simulink model "Test9"  (R2021a)
settings: Solver=FixedStepDiscrete  StartTime=0.0  StopTime=tsim  FixedStep=Ts  RelTol=1e-3  EnableMultiTasking=on
InitFcn:
  | Fs = 2048; Ts = 1/Fs;tsim = inf;
undefined symbols (not defined in the file or in its folder): DiscIntNeverNeededParam
libraries: sperte_lib x24, simulink x5, Quintic_Polynomial_Trajectory_Library x3, raspberrypiCommlib x2
(part 2 of 2)

== system Test9/RobotArm/Supervisor/Supervisory Controller Z/Selector1 ==
  In1 : Inport
  Demux2 : Demux  Outputs=3
  Terminator4 : Terminator
  Terminator5 : Terminator
  Out1 : Outport
  wires:
  Demux2/3 -> Out1/1
  Demux2/2 -> Terminator5/1
  In1/1 -> Demux2/1
  Demux2/1 -> Terminator4/1

== system Test9/RobotArm/Supervisor/Supervisory Controller Z/Selector2 ==
  In1 : Inport
  Demux2 : Demux  Outputs=3
  Terminator4 : Terminator
  Terminator5 : Terminator
  Out1 : Outport
  wires:
  Demux2/1 -> Terminator4/1
  In1/1 -> Demux2/1
  Demux2/2 -> Terminator5/1
  Demux2/3 -> Out1/1

== system Test9/RobotArm/Supervisor/Supervisory Controller Z/Selector3 ==
  In1 : Inport
  Demux2 : Demux  Outputs=3
  Terminator5 : Terminator
  Out1 : Outport
  Out2 : Outport  Port=2
  wires:
  Demux2/3 -> Out1/1
  Demux2/2 -> Terminator5/1
  In1/1 -> Demux2/1
  Demux2/1 -> Out2/1

== system Test9/RobotArm/Supervisor/Supervisory Conveyor/Controller Conveyor ==
  Input : Inport
  Dct1lowpass : sperte_lib/Dct1lowpass  f_den=30
      settings: SourceProductName=SPERTE project library
  Dctintegrator3 : S-Function  FunctionName=dweakint  Parameters=f_num, 0.001  SFunctionDeploymentMode=off  EnableBusSupport=off  mask(dctools){f_num=0.01}
      mask prompts: f_num "Zero [Hz]"
      mask help: This block implements a discrete time weak integrator filter.
      mask Display: disp('DCT integrator')
  Dctleadlag : sperte_lib/Dctleadlag  f_num=3  f_den=20
      settings: SourceProductName=SPERTE project library
  Gain1 : Gain  Gain=10*2.5/500
  Output : Outport
  wires:
  Input/1 -> Gain1/1
  Dctintegrator3/1 -> Dct1lowpass/1
  Dctleadlag/1 -> Output/1
  Gain1/1 -> Dctintegrator3/1
  Dct1lowpass/1 -> Dctleadlag/1

== system Test9/RobotArm/Supervisor/Subsystem/LED Ring/Subsystem ==
  note: U(k)
  note: Edge
  U : Inport
  Delay : Delay  DelayLength=1  InitialCondition=0
  NOT : Logic  Operator=NOT  IconShape=distinctive  AllPortsSameDT=off  OutDataTypeStr=boolean
  String Compare : StringCompare
  Y : Outport  InitialOutput=0
  wires:
  Delay/1 -> String Compare/2  "U(k-1)"
  String Compare/1 -> NOT/1
  NOT/1 -> Y/1
  U/1 -> Delay/1, String Compare/1

== system Test9/RobotArm/Supervisor/Subsystem/LED Ring/Subsystem3 ==
  In1 : Inport
  Enable : EnablePort
  If : If  IfExpression=u1 == 1
  If Action Subsystem : Subsystem  TreatAsAtomicUnit=on
  If Action Subsystem1 : Subsystem  TreatAsAtomicUnit=on
  OR : Logic  Operator=OR  IconShape=distinctive  AllPortsSameDT=off  OutDataTypeStr=boolean
  String Compare : StringCompare
  String Compare1 : StringCompare
  String Constant1 : StringConstant  String='black'
  String Constant4 : StringConstant  String='white'
  wires:
  If/1 -> If Action Subsystem/Action
  String Compare/1 -> OR/1
  String Constant4/1 -> String Compare/2
  In1/1 -> If Action Subsystem1/1(In1), String Compare1/1, String Compare/1, If Action Subsystem/1(In1)
  If/2 -> If Action Subsystem1/Action
  OR/1 -> If/1
  String Compare1/1 -> OR/2
  String Constant1/1 -> String Compare1/2

== system Test9/RobotArm/Supervisor/Subsystem/LED Ring/Subsystem3/If Action Subsystem ==
  In1 : Inport
  Action Port : ActionPort  ActionPortLabel=if(u1 == 1)
  Constant1 : Constant  Value=13  OutDataTypeStr=uint8
  Matrix Concatenate1 : Concatenate  ConcatenateDimension=2
  Serial Write1 : raspberrypiCommlib/Serial Write  board=Pi 4 Model B  SCIModule_=/dev/ttyACM0  Baudrate_=9600  Parity=None  StopBits_=1  HardwareFlowControl=None  ByteOrder=LittleEndian  OutputStatus=off  blockPlatform=RaspberryPi
      settings: SourceProductBaseCode=RASPPI
  String to ASCII1 : StringToASCII
  wires:
  In1/1 -> String to ASCII1/1
  String to ASCII1/1 -> Matrix Concatenate1/1
  Matrix Concatenate1/1 -> Serial Write1/1
  Constant1/1 -> Matrix Concatenate1/2

== system Test9/RobotArm/Supervisor/Subsystem/LED Ring/Subsystem3/If Action Subsystem1 ==
  In1 : Inport
  Action Port : ActionPort  ActionPortLabel=else
  Constant : Constant  Value=13  OutDataTypeStr=uint8
  Matrix Concatenate : Concatenate  ConcatenateDimension=2
  Serial Write : raspberrypiCommlib/Serial Write  board=Pi 4 Model B  SCIModule_=/dev/ttyACM0  Baudrate_=9600  Parity=None  StopBits_=1  HardwareFlowControl=None  ByteOrder=LittleEndian  OutputStatus=off  blockPlatform=RaspberryPi
      settings: SourceProductBaseCode=RASPPI
  String Concatenate : StringConcatenate
  String Constant3 : StringConstant  String='color '
  String to ASCII : StringToASCII
  wires:
  Matrix Concatenate/1 -> Serial Write/1
  String to ASCII/1 -> Matrix Concatenate/1
  String Concatenate/1 -> String to ASCII/1
  String Constant3/1 -> String Concatenate/1
  Constant/1 -> Matrix Concatenate/2
  In1/1 -> String Concatenate/2

== matlab function Test9/RobotArm/Supervisor/Supervisory Controller R/Angle2Z ==
  data: u input; y output
function y = fcn(u)

% Z and X angles to height of the robotarm. The initial angles are the
% angles from the horizontal line to the correponding arm.

initialanglez = 0.6150;
initialanglex = (75.3841/180)*pi;
thetax = -u(2)+initialanglex;
thetaz = u(3)+initialanglez;

theta1 = thetax;
theta2 = thetaz;

% parameters

l1 = 80e-3;
l2 = 130e-3;
l3 = 165e-3;
l4 = 130e-3;
l5 = 120e-3;
l6 = 120e-3 + 65e-3;
length_head = 45e-3;
l7 = 81e-3;

% functions

fx1 = l1*cos(theta1);
fy1 = l1*sin(theta1);

fx2 = l2*cos(theta2);
fy2 = l3 + l2*sin(theta2);

d12 = sqrt((fx2 - fx1)^2 + (fy2 - fy1)^2);
d13 = sqrt(fx1^2 + (l3 - fy1)^2);

phi1 = acos((l2^2 + d12^2 -d13^2)/(2*d12*l2));
phi2 = acos((l5^2 + d12^2 -l4^2)/(2*d12*l5));

yf = fy2- l6*sin(pi - phi1 - phi2 - theta2);

y = yf-length_head+l7;

== matlab function Test9/RobotArm/Supervisor/Supervisory Controller Z/Angle2Z ==
  data: u input; y output
function y = fcn(u)

% Z and X angles to height of the robotarm. The initial angles are the
% angles from the horizontal line to the correponding arm.

initialanglez = 0.6150;
initialanglex = (75.3841/180)*pi;
thetax = -u(2)+initialanglex;
thetaz = u(3)+initialanglez;

theta1 = thetax;
theta2 = thetaz;

% parameters

l1 = 80e-3;
l2 = 130e-3;
l3 = 165e-3;
l4 = 130e-3;
l5 = 120e-3;
l6 = 120e-3 + 65e-3;
length_head = 45e-3;
l7 = 81e-3;

% functions

fx1 = l1*cos(theta1);
fy1 = l1*sin(theta1);

fx2 = l2*cos(theta2);
fy2 = l3 + l2*sin(theta2);

d12 = sqrt((fx2 - fx1)^2 + (fy2 - fy1)^2);
d13 = sqrt(fx1^2 + (l3 - fy1)^2);

phi1 = acos((l2^2 + d12^2 -d13^2)/(2*d12*l2));
phi2 = acos((l5^2 + d12^2 -l4^2)/(2*d12*l5));

yf = fy2- l6*sin(pi - phi1 - phi2 - theta2);

y = yf-length_head+l7;

== stateflow chart Test9/Controller/Stateflow  ==
  settings: updateMethod=DISCRETE  sampleTime=0.00048828125  executeAtInitialization=1
  state Robot_Arm [parallel]
    settings: executionOrder=4
    state Start_Home
      entry:
      [R_rad, X_rad, Z_rad] = invkin(X_home, Y_home, Z_home); %Move to home
      WaitFor = TimeToMoveCalc(TimeBuffer, R_radVavg, X_radVavg, Z_radVavg, R_rad, X_rad, Z_rad, R_radMeasure, X_radMeasure, Z_radMeasure)
    state Await_Scanning
      entry:
      ScanAgain
      PumpOff
    state Move_TrackingAwaitingLocation
      entry:
      [R_rad, X_rad, Z_rad] = invkinBound(X_in, Y_StartMoveAlong , Z_StartMoveAlong);
      WaitFor = TimeToMoveCalc(TimeBuffer, R_radVavg, X_radVavg, Z_radVavg, R_rad, X_rad, Z_rad, R_radMeasure, X_radMeasure, Z_radMeasure)
    state Get_Data
      entry:
      Y_data = Y_in;
      X_data = X_in;
      Z_arm = Z_StartMoveAlong; %99 or Z_home
      Area_data = Area_in;
    state Move_TrackingAndPickUp
      entry:
      if (n<1)
      Y_obj = Y_data + (TimeStep+CameraDelay)*Conveyor;
      n = n+1;
      elseif (n>=1)
      Y_obj = Y_obj+(TimeStep)*Conveyor;
      %if Y_obj <= Y_StartMoveAlong %-60
      % [R_rad, X_rad, Z_rad] = invkinBound(X_data, Y_obj, Z_arm)
      if Y_obj > Y_StartLowering %-60
      Z_arm = Z_arm - abs(Z_StartMoveAlong-Z_PickUpHeight)/abs(Y_PickUpAt-Y_StartLowering)*Conveyor*TimeStep;
      [R_rad, X_rad, Z_rad] = invkinBound(X_data, Y_obj, Z_arm);
      if Z_arm <= Z_PickUpHeight % 80
      Tracking = false;
      send(VacuumOn,Pump_stateflow);
      end
      end
      end
    state Move_toGoalHeight1
      entry:
      Z_arm = Z_arm+18;
      [R_radt, X_radt, Z_radt] = invkinBound(X_data, Y_obj, Z_arm); %Move to goal xy at setpoint height
      WaitFor = TimeToMoveCalc(TimeBuffer, R_radVavg, X_radVavg, Z_radVavg, R_radt, X_radt, Z_radt, R_radMeasure, X_radMeasure, Z_radMeasure)
    state Move_toGoalHeight2
      entry:
      [R_radt, X_radt, Z_radt] = invkinBound(150, 60, Z_arm+2); %Move to goal xy at setpoint height
      WaitFor = TimeToMoveCalc(TimeBuffer, R_radVavg, X_radVavg, Z_radVavg, R_radt, X_radt, Z_radt, R_radMeasure, X_radMeasure, Z_radMeasure)
    state Move_toGoalLower
      entry:
      GetEndXY
      [R_rad, X_rad, Z_rad] = invkinBound(EndX, EndY, Z_arm+2); %Lower until ready to drop item
      WaitFor = TimeToMoveCalc(TimeBuffer, R_radVavg, X_radVavg, Z_radVavg, R_rad, X_rad, Z_rad, R_radMeasure, X_radMeasure, Z_radMeasure)
    state Eject_object
      entry:
      BlowOn
    (default) -> Start_Home
    (junction 408) -> Start_Home
    Eject_object -> (junction 408) : [VacuumSensor>-0.014]
    Start_Home -> Await_Scanning : [after(WaitFor,sec)]
    Await_Scanning -> Move_TrackingAwaitingLocation : [Area_in>=2000]
    Move_TrackingAwaitingLocation -> Get_Data : [(after(WaitFor, sec))&&(Y_in> -120)]{Tracking = true, n=0}
    Get_Data -> Move_TrackingAndPickUp
    Move_TrackingAndPickUp -> Move_TrackingAndPickUp [order 1] : [Tracking == true&&after(TimeStep,sec)]
    Move_TrackingAndPickUp -> Move_toGoalHeight1 [order 2] : [(Tracking==false)&&(VacuumSensor<-0.35)]
    Move_toGoalHeight1 -> Move_toGoalHeight2 : [after(WaitFor, sec)]
    Move_toGoalHeight2 -> Move_toGoalLower : [after(WaitFor, sec)]
    Move_toGoalLower -> Eject_object : [after(WaitFor, sec)]
  state Object_Detection [parallel]
    settings: executionOrder=1
    state Seeking
      entry:
    state AwaitSeeking
      entry:
      GetProduct
    state ProvideData
      entry:
      if (3000<=Area_data)&&(Area_data<6000)
      nPawn = nPawn + 1;
      EndX = 45-(nPawn-1)*48; % Pawn (a-h)2
      EndY = 193;
      elseif (6000<=Area_data)&&(Area_data<8600)
      EndX = -51; % Knight b1
      EndY = 145;
      elseif (8600<=Area_data)&&(Area_data<12000)
      EndX = -3; % Bishop c1
      EndY = 145;
      elseif (12000<=Area_data)&&(Area_data<15000)
      EndX = -98; % Rook a1
      EndY = 145;
      elseif (15000<=Area_data)&&(Area_data<17000)
      EndX = 45; % Queen d1
      EndY = 145;
      elseif (17000<=Area_data)&&(Area_data<27000)
      EndX = 45; % King d1 (there is no e1)
      EndY = 145;
      end
    (default) -> Seeking
    (junction 428) -> Seeking
    (junction 448) -> (junction 428)
    Seeking -> AwaitSeeking : [Area_in>=2000]
    AwaitSeeking -> ProvideData : GetEndXY
    ProvideData -> (junction 448) : ScanAgain
  state Pump_stateflow [parallel]
    settings: executionOrder=3
    state Pump_off
      during:
      Pump = 0 %Bar
      Blow_suck = 1
    state Vacuum
      during:
      Pump = -1 %Bar
      Blow_suck = 0
    state Blow
      during:
      Pump = 1 %Bar
      Blow_suck = 1
    (default) -> Pump_off
    Pump_off -> Vacuum [order 1] : VacuumOn
    Vacuum -> Pump_off [order 1] : PumpOff
    Blow -> Pump_off [order 2] : PumpOff
    Pump_off -> Blow [order 2] : BlowOn
    Blow -> Vacuum [order 1] : VacuumOn
    Vacuum -> Blow [order 2] : BlowOn
  state Belt [parallel]
    settings: executionOrder=2
    state Belt_Home
      during:
      Conveyor = 30;
    (default) -> Belt_Home
  data: errorAngleDegree function_input; R_rad_GoTo function_input; X_rad_GoTo function_input; Z_rad_GoTo function_input; R_rad_Current function_input; X_rad_Current function_input; Z_rad_Current function_input; RXZ_OnPosition function_output; x_kin function_input; y_kin function_input; z_kin function_input; PsikinBound function_output; PhikinBound function_output; ThetakinBound function_output; x_kin function_input; y_kin function_input; z_kin function_input; Psikin function_output; Phikin function_output; Thetakin function_output; BufferTime function_input; Rrad_Vavg function_input; Xrad_Vavg function_input; Zrad_Vavg function_input; Rrad_goto function_input; Xrad_goto function_input; Zrad_goto function_input; Rrad_current function_input; Xrad_current function_input; Zrad_current function_input; MoveAfterXSec function_output; R_rad output; X_in input; X_rad output; Z_rad output; Y_in input; Area_in input; VacuumSensor input; Blow_suck output; Conveyor output; Pump output; Tracking output boolean =true; R_radMeasure input; X_radMeasure input; Z_radMeasure input; R_radVavg input; X_radVavg input; Z_radVavg input; WaitFor local; CameraDelay input; Y_StartMoveAlong local =-60; Y_StartLowering local =-60; Z_PickUpHeight local =80; X_home local =160; Y_home local =0; Z_home local =90; Z_StartMoveAlong local =90; Y_PickUpAt local =0; nPawn local =0; X_data local; Y_data local; EndX local; EndY local; TimeBuffer local =0.4; n local =0; TimeStep local =0.01; R_radt local; X_radt local; Z_radt local; Y_obj local =0; Z_arm local =90; Area_data local =0
  events: GetProduct local FUNCTION_CALL_EVENT; ScanAgain local FUNCTION_CALL_EVENT; VacuumOn local FUNCTION_CALL_EVENT; BlowOn local FUNCTION_CALL_EVENT; PumpOff local FUNCTION_CALL_EVENT; GetEndXY local RISING_EDGE_EVENT
  function RXZ_OnPosition = RXZOnPosition(errorAngleDegree, R_rad_GoTo, X_rad_GoTo, Z_rad_GoTo, R_rad_Current, X_rad_Current, Z_rad_Current):
    | function RXZ_OnPosition = RXZOnPosition(errorAngleDegree, R_rad_GoTo, X_rad_GoTo, Z_rad_GoTo, R_rad_Current, X_rad_Current, Z_rad_Current)
    | 
    | % Standard Output
    | OnPositionR = false;
    | OnPositionX = false;
    | OnPositionZ = false;
    | RXZ_OnPosition = false;
    | 
    | % Calculate error
    | R_error = abs(R_rad_Current-R_rad_GoTo);
    | X_error = abs(X_rad_Current-X_rad_GoTo);
    | Z_error = abs(Z_rad_Current-Z_rad_GoTo);
    | errorAngleRad = errorAngleDegree;
    | 
    | 
    | % Check if error is within a certain percentage of the current movement
    | if (R_error <= errorAngleRad)
    |     OnPositionR = true;
    | end
    | if (X_error <= errorAngleRad)
    |     OnPositionX = true;
    | end
    | if (X_error <= errorAngleRad)
    |     OnPositionZ = true;
    | end
    | % Return function as true when final coordinates are reached for all
    | if OnPositionR&&OnPositionX&&OnPositionZ
    |     RXZ_OnPosition = true;
    | end
    | 
    | 
    | end
  function [PsikinBound, PhikinBound, ThetakinBound] = invkinBound(x_kin, y_kin, z_kin):
    | function [PsikinBound, PhikinBound, ThetakinBound] = invkinBound(x_kin, y_kin, z_kin)
    | %% function to determine the angle of the motors for the right x,y,z position
    | %% Psi is angle R motor in rad
    | %% Phi is angle X motor in rad
    | %% Theta is angle Z motor in rad
    | %% x [mm] is perpendicular to the conveyer
    | %% y [mm] is in the direction of the conveyer
    | %% Z [mm]is the height from the conveyer
    | 
    | % These offsets are for the homing position (160, 0, 99) w.r.t. the middle
    | % of the robotarm on the table
    | r_offset = 0;
    | x_offset = -0.2551;
    | z_offset = -0.6150;
    | 
    | mm  = 10^(-3);
    | L1  = 130*mm;
    | L2a = 120*mm;
    | L2b = 65*mm;
    | L2  = L2a+L2b;
    | L3  = 80*mm;
    | L4  = 130*mm;
    | ED  = 165*mm;
    | OE  = 81*mm;
    | 
    | %% measurements
    | length_head = 45*mm;              % length of the vacuum head
    | height_conveyer = 0*mm;           % height of the conveyer
    | X0 = 0*mm;                        % distance center robot to conveyer
    | Y0      =   0*mm;                    % distance center plate to grid
    | 
    | %% Determine the x, y and z coordinates of the grid in [m]
    | Y = Y0+y_kin*mm;
    | X = X0+x_kin*mm;
    | Z = length_head+height_conveyer+z_kin*mm;
    | 
    | %% Psi - motor R
    | R   =   sqrt(X^2+Y^2);
    | PsikinBound =   atan2(Y,X);
    | 
    | %% Theta - motor Z
    | L_DB    = sqrt(R^2+(OE+ED-Z)^2);
    | H_GDB   = asin(R/L_DB);
    | H_CDB   = acos((L1^2+L_DB^2-L2^2)/(2*L1*L_DB));
    | ThetakinBound   = H_CDB+H_GDB-.5*pi;
    | 
    | %% PHI - motor X
    | H_DBC   = acos((L2^2+L_DB^2-L1^2)/(2*L2*L_DB));
    | H_DCB   = pi-H_CDB-H_DBC;
    | L_DF    = sqrt(L1^2+L2a^2-2*L1*L2a*cos(H_DCB));
    | H_CDF   = acos((L1^2+L_DF^2-L2a^2)/(2*L1*L_DF));
    | H_EDF   = H_CDB+H_GDB-H_CDF;
    | L_EF    = sqrt(L_DF^2+ED^2-2*L_DF*ED*cos(H_EDF));
    | H_DEF   = acos((L_EF^2+ED^2-L_DF^2)/(2*L_EF*ED));
    | Phi_2   = acos((L3^2+L_EF^2-L4^2)/(2*L3*L_EF));
    | Phi_1   = 0.5*pi-H_DEF;
    | PhikinBound     = Phi_1+Phi_2;
    | 
    | %% Final results of the angles
    | PsikinBound     = PsikinBound+r_offset;      % offset R
    | PhikinBound     = pi/2-PhikinBound+x_offset; % offset X
    | ThetakinBound   = ThetakinBound+z_offset;    % offset Z
    | 
    | % Check if answer is real, otherwise take sign of imaginary for rotation
    | % Set answer so it is real and definitely out of bounds, but with right sign 
    | if ~isreal(PsikinBound)
    | PsikinBound = sign(imag(PsikinBound))*6;
    | end
    | if ~isreal(PhikinBound)
    | PhikinBound = sign(imag(PhikinBound))*6;
    | end
    | if ~isreal(ThetakinBound)
    | ThetakinBound = sign(imag(ThetakinBound))*6;
    | end
    | 
    | % Check if angle is within bound, otherwise take the boundary
    | if ~((PsikinBound>-1)&&(PsikinBound<2))
    |     PsikinBound = min(max(PsikinBound,-1),2);
    | end
    | if ~((PhikinBound>-0.5)&&(PhikinBound<0.5))
    |     PhikinBound = min(max(PhikinBound,-0.5),0.5);
    | end
    | if ~((ThetakinBound>-0.3)&&(ThetakinBound<0.2))
    |     ThetakinBound = min(max(ThetakinBound,-0.3),0.2);
    | end
    | 
    | end
  function [Psikin, Phikin, Thetakin] = invkin(x_kin, y_kin, z_kin):
    | function [Psikin, Phikin, Thetakin] = invkin(x_kin, y_kin, z_kin)
    | %% function to determine the angle of the motors for the right x,y,z position
    | %% Psi is angle R motor in rad
    | %% Phi is angle X motor in rad
    | %% Theta is angle Z motor in rad
    | %% x [mm] is perpendicular to the conveyer
    | %% y [mm] is in the direction of the conveyer
    | %% Z [mm]is the height from the conveyer
    | 
    | % These offsets are for the homing position (160, 0, 99) w.r.t. the middle
    | % of the robotarm on the table
    | r_offset = 0;
    | x_offset = -0.2551;
    | z_offset = -0.6150;
    | 
    | mm  = 10^(-3);
    | L1  = 130*mm;
    | L2a = 120*mm;
    | L2b = 65*mm;
    | L2  = L2a+L2b;
    | L3  = 80*mm;
    | L4  = 130*mm;
    | ED  = 165*mm;
    | OE  = 81*mm;
    | 
    | %% measurements
    | length_head = 45*mm;              % length of the vacuum head
    | height_conveyer = 0*mm;           % height of the conveyer
    | X0 = 0*mm;                        % distance center robot to conveyer
    | Y0      =   0*mm;                    % distance center plate to grid
    | 
    | %% Determine the x, y and z coordinates of the grid in [m]
    | Y = Y0+y_kin*mm;
    | X = X0+x_kin*mm;
    | Z = length_head+height_conveyer+z_kin*mm;
    | 
    | %% Psi - motor R
    | R   =   sqrt(X^2+Y^2);
    | Psikin =   atan2(Y,X);
    | 
    | %% Theta - motor Z
    | L_DB    = sqrt(R^2+(OE+ED-Z)^2);
    | H_GDB   = asin(R/L_DB);
    | H_CDB   = acos((L1^2+L_DB^2-L2^2)/(2*L1*L_DB));
    | Thetakin   = H_CDB+H_GDB-.5*pi;
    | 
    | %% PHI - motor X
    | H_DBC   = acos((L2^2+L_DB^2-L1^2)/(2*L2*L_DB));
    | H_DCB   = pi-H_CDB-H_DBC;
    | L_DF    = sqrt(L1^2+L2a^2-2*L1*L2a*cos(H_DCB));
    | H_CDF   = acos((L1^2+L_DF^2-L2a^2)/(2*L1*L_DF));
    | H_EDF   = H_CDB+H_GDB-H_CDF;
    | L_EF    = sqrt(L_DF^2+ED^2-2*L_DF*ED*cos(H_EDF));
    | H_DEF   = acos((L_EF^2+ED^2-L_DF^2)/(2*L_EF*ED));
    | Phi_2   = acos((L3^2+L_EF^2-L4^2)/(2*L3*L_EF));
    | Phi_1   = 0.5*pi-H_DEF;
    | Phikin     = Phi_1+Phi_2;
    | 
    | %% Final results of the angles
    | Psikin     = Psikin+r_offset;      % offset R
    | Phikin     = pi/2-Phikin+x_offset; % offset X
    | Thetakin   = Thetakin+z_offset;    % offset Z
    | end
  function MoveAfterXSec = TimeToMoveCalc(BufferTime, Rrad_Vavg, Xrad_Vavg, Zrad_Vavg, Rrad_goto, Xrad_goto, Zrad_goto, Rrad_current, Xrad_current, Zrad_current):
    | function  MoveAfterXSec = TimeToMoveCalc(BufferTime, Rrad_Vavg, Xrad_Vavg, Zrad_Vavg, Rrad_goto, Xrad_goto, Zrad_goto, Rrad_current, Xrad_current, Zrad_current)
    | 
    | %TimeBuffer = 0.4; %sec
    | %Rrad_Vavg = 1;
    | %Xrad_Vavg = 1;
    | %Zrad_Vavg = 1;
    | %Rrad_goto = 2;
    | %Xrad_goto = 0.5;
    | %Zrad_goto = 0.2;
    | %Rrad_current = -1;
    | %Xrad_current = -0.5;
    | %Zrad_current = -0.3;
    | 
    | 
    | % t = delta_x/v_avg
    | Rrad_movetime = abs(Rrad_goto - Rrad_current)/Rrad_Vavg; 
    | Xrad_movetime = abs(Xrad_goto - Xrad_current)/Xrad_Vavg; 
    | Zrad_movetime = abs(Zrad_goto - Zrad_current)/Zrad_Vavg; 
    | 
    | 
    | 
    | MoveAfterXSec = BufferTime + max([Rrad_movetime, Xrad_movetime, Zrad_movetime]);
    | 
    | 
    | 
    | 
    | end

== stateflow chart Test9/RobotArm/Supervisor/Supervisory Conveyor/Supervisor ==
  state Waiting
    %Homing has to wait for 3 sec
    %as the new arm gets the 5V enable signal
    %after pressing start to avoi d moving to X0 too
    %early
  state Homing
    entry:
    %Set jog speed and homing state
    Ready=0;
    homingBusy = 1;
    jogSpeed = 20;
    homeControllerEnabled=1;
  state MovetoX0
    entry:
    jogSpeed = -20;
  state CheckRobotIsON
    entry:
    jogSpeed = 0;
  state WaitForRest
    entry: Ready = 1;
  state EnableRunAndSafety
    entry:
    resetEnc=0;
    homingBusy=0;
  state ResetEnc
    entry:
    resetEnc=1;
    homeControllerEnabled=0;
  (default) -> Waiting
  Waiting -> Homing : after(1,sec)
  Homing -> MovetoX0 : after(3,sec)
  MovetoX0 -> CheckRobotIsON : %Allow time for moving
      | after(3,sec)
  CheckRobotIsON -> WaitForRest : after(1,sec)
  WaitForRest -> ResetEnc : [AllReady]
  ResetEnc -> EnableRunAndSafety : after(1,sec)
  data: jogSpeed output double; homeControllerEnabled output double; resetEnc output double; homingBusy output double =1; Ready output double =1; AllReady input boolean; StopSim output double =0

== stateflow chart Test9/RobotArm/Supervisor/Supervisory Controller R/Supervisor ==
  state Waiting
    %Homing has to wait for 3 sec
    %as the new arm gets the 5V enable signal
    %after pressing start to avoid moving to X0 too
    %early
    Ready=0;
    toPoint = 0;
    homingBusy = 1;
    jogSpeed = -0.001;
    homeControllerEnabled=0.01;
  state Waiting1
    %Homing has to wait for 3 sec
    %as the new arm gets the 5V enable signal
    %after pressing start to avoid moving to X0 too
    %early
    Ready=0;
    toPoint = 0;
    homingBusy = 1;
    jogSpeed = 0;
    homeControllerEnabled=1;
  state AirbagLeft
    entry:
    homingBusy = 1;
    currentcarPos = carPos;
    airBagEnabled = 1;
    airBagRef=currentcarPos+0.02;
  state DisableOutputs
    entry:
    controlEnabled=0;
    StopSim = 1;
  state Homing
    entry:
    %Set jog speed and homing state
    Ready=0;
    toPoint = 0;
    homingBusy = 1;
    jogSpeed = -0.4;
    homeControllerEnabled=1;
  state AirbagLeft1
    entry:
    homingBusy = 1;
    currentcarPos = carPos;
    airBagEnabled = 1;
    airBagRef=currentcarPos-0.02;
  state AirbagConveyor
    entry:
    homingBusy = 1;
    currentcarPos = carPos;
    airBagEnabled = 1;
    airBagRef=currentcarPos+0.02
  state MovetoX0
    entry:
    jogSpeed = 0.0;
    toPoint = Offset_homing
  state STOPRobotIsOFF
    entry:
    StopSim=1;
  state CheckRobotIsON
  state EnableRunAndSafety
    entry:
    resetEnc=0;
    homingBusy=0;
  state RobotIsON
  state WaitForRest
    entry: Ready = 1;
  state ResetEnc
    entry:
    homingBusy = 100;
    resetEnc=1;
    homeControllerEnabled=0;
  (default) -> Waiting
  Waiting -> Waiting1 : after(1,sec)
  Waiting1 -> Homing : after(3,sec)
  AirbagLeft -> DisableOutputs : after(3,sec)
  AirbagConveyor -> DisableOutputs : after(3,sec)
  AirbagLeft1 -> DisableOutputs : after(3,sec)
  EnableRunAndSafety -> AirbagLeft [order 2] : [carPos<-1.1]
  Homing -> MovetoX0 : %Transition if homeswitch becomes high
      | [homeSwitch]
  EnableRunAndSafety -> AirbagLeft1 [order 1] : [carPos>2.7]
  EnableRunAndSafety -> AirbagConveyor [order 3] : [zcoordinate<0.056&&carPos < 1.3]
  MovetoX0 -> CheckRobotIsON [order 2] : % Allow time for moving
      | after(5,sec)
  MovetoX0 -> CheckRobotIsON [order 1] : [carPos == toPoint]
  CheckRobotIsON -> STOPRobotIsOFF [order 1] : [carPos<-3]
  CheckRobotIsON -> RobotIsON [order 2]
  RobotIsON -> WaitForRest : after(1,sec)
  ResetEnc -> EnableRunAndSafety : after(1,sec)
  WaitForRest -> ResetEnc : [AllReady]
  data: jogSpeed output double; toPoint output double; homeControllerEnabled output double; resetEnc output double; homingBusy output double =1; homeSwitch input boolean; carPos input double; airBagEnabled output double =0; airBagRef output double =0; controlEnabled output double =1; Ready output double =1; AllReady input boolean; StopSim output double =0; zcoordinate input; currentcarPos local double; Offset_homing input

== stateflow chart Test9/RobotArm/Supervisor/Supervisory Controller X/Supervisor ==
  state Waiting
    %Homing has to wait for 3 sec
    %as the new arm gets the 5V enable signal
    %after pressing start to avoid moving to X0 too
    %early
    Ready=0;
    toPoint = 0;
    homingBusy = 1;
    jogSpeed = -0.001;
    homeControllerEnabled=0.01;
  state DisableOutputs
    entry:
    controlEnabled=0;
    StopSim=1;
  state AirbagLeft
    entry:
    homingBusy = 1;
    currentcarPos = carPos;
    airBagEnabled = 1;
    airBagRef=currentcarPos+0.02;
  state Waiting1
    %Homing has to wait for 3 sec
    %as the new arm gets the 5V enable signal
    %after pressing start to avoid moving to X0 too
    %early
    Ready=0;
    toPoint = 0;
    homingBusy = 1;
    jogSpeed = 0;
    homeControllerEnabled=1;
  state AirbagRight
    entry:
    homingBusy = 1;
    currentcarPos = carPos;
    airBagEnabled = 1;
    airBagRef=currentcarPos-0.02;
  state Homing
    entry:
    %Set jog speed and homing state
    jogSpeed = -0.2;
    homeControllerEnabled=1;
  state MovetoX0
    entry:
    jogSpeed = 0.0;
    toPoint = offset_homing;
  state EnableRunAndSafety
    entry:
    resetEnc=0;
    homingBusy=0;
  state WaitForRest
    entry: Ready = 1;
  state ResetEnc
    entry:
    resetEnc=1;
    homeControllerEnabled=0;
  (default) -> Waiting
  Waiting -> Waiting1 : after(2,sec)
  AirbagLeft -> DisableOutputs : after(3,sec)
  AirbagRight -> DisableOutputs : after(3,sec)
  EnableRunAndSafety -> AirbagLeft [order 1] : [carPos<-0.5]
  Waiting1 -> Homing : after(3,sec)
  EnableRunAndSafety -> AirbagRight [order 2] : [carPos>1.1 ]
  Homing -> MovetoX0 : %Transition if homeswitch becomes high
      | [homeSwitch]
  MovetoX0 -> WaitForRest [order 2] : %Allow time for moving
      | after(5,sec)
  MovetoX0 -> WaitForRest [order 1] : [carPos == toPoint]
  ResetEnc -> EnableRunAndSafety : after(1,sec)
  WaitForRest -> ResetEnc : [AllReady]
  data: jogSpeed output double; toPoint output double; homeControllerEnabled output double; resetEnc output double; homingBusy output double =1; homeSwitch input boolean; carPos input double; airBagEnabled output double =0; airBagRef output double =0; controlEnabled output double =1; Ready output double =1; AllReady input boolean; StopSim output double =0; currentcarPos local double; offset_homing input

== stateflow chart Test9/RobotArm/Supervisor/Supervisory Controller Z/Supervisor ==
  state Waiting
    %Homing has to wait for 3 sec
    %as the new arm gets the 5V enable signal
    %after pressing start to avoid moving to X0 too
    %early
    Ready=0;
    toPoint = 0;
    homingBusy = 1;
    jogSpeed = 0.001;
    homeControllerEnabled=0.1;
  state Waiting1
    %Homing has to wait for 3 sec
    %as the new arm gets the 5V enable signal
    %after pressing start to avoid moving to X0 too
    %early
    Ready=0;
    toPoint = 0;
    jogSpeed =  0 ;
    homeControllerEnabled=1;
  state DisableOutputs
    entry:
    controlEnabled=0;
    StopSim=1;
  state Homing
    entry:
    %Set jog speed and homing state
    toPoint = 0;
    Ready = 0;
    homingBusy = 1;
    jogSpeed = 0.2;
    homeControllerEnabled=1;
  state AirbagConveyor
    entry:
    homingBusy = 1;
    currentcarPos = carPos;
    airBagEnabled = 1;
    airBagRef=currentcarPos+0.1
  state MovetoX0
    entry:
    jogSpeed = 0.0;
    toPoint = offset_homing;
  state AirbagTop
    entry:
    homingBusy = 1;
    currentcarPos = carPos;
    airBagEnabled = 1;
    airBagRef=currentcarPos-0.02;
  state WaitForRest
    entry: Ready = 1;
  state EnableRunAndSafety
    entry:
    resetEnc=0;
    homingBusy=0;
  state AirbagDrop
    entry:
    homingBusy = 1;
    currentcarPos = carPos;
    airBagEnabled = 1;
    airBagRef=currentcarPos+0.02
  state ResetEnc
    entry:
    resetEnc=1;
    homeControllerEnabled=0;
    Ready = 1;
  (default) -> Waiting
  Waiting -> Waiting1 : after(2,sec)
  Waiting1 -> Homing : after(2,sec)
  AirbagDrop -> DisableOutputs : after(3,sec)
  AirbagConveyor -> DisableOutputs : after(3,sec)
  AirbagTop -> DisableOutputs : after(3,sec)
  EnableRunAndSafety -> AirbagConveyor [order 1] : [zcoordinate<0.056&&rcoordinate < 1.3]
  Homing -> MovetoX0 : %Transition if homeswitch becomes high
      | [homeSwitch]
  EnableRunAndSafety -> AirbagTop [order 2] : [carPos>0.3]
  MovetoX0 -> WaitForRest [order 2] : %Allow time for moving
      | after(5,sec)
  MovetoX0 -> WaitForRest [order 1] : [carPos == toPoint]
  WaitForRest -> ResetEnc : [AllReady]
  EnableRunAndSafety -> AirbagDrop [order 3] : [zcoordinate<0&&rcoordinate>1.3]
  ResetEnc -> EnableRunAndSafety : after(1,sec)
  data: jogSpeed output double; toPoint output double; homeControllerEnabled output double; resetEnc output double; homingBusy output double =1; homeSwitch input boolean; carPos input double; airBagEnabled output double =0; airBagRef output double =0; controlEnabled output double =1; Ready output double =1; AllReady input boolean; StopSim output double =0; zcoordinate input double; currentcarPos local double; rcoordinate input double; offset_homing input
